simulink model "Riccati_Simulation"  (R2016b)
settings: Solver=VariableStepAuto  StartTime=0.0  StopTime=120  RelTol=1e-1
values from neighbouring files (symbols this model uses):
  A1k = [A1s                     E_w*C_w ... (first row only)    [RiccatiBerechnung_Anlage.m]    (also in RiccatiBerechnunguPlot_Simulation.m)
  A2k = [A2                     E2*C2_s ... (first row only)    [RiccatiBerechnung_Anlage.m]    (also in RiccatiBerechnunguPlot_Simulation.m)
  Ak = [A1                      E*C_s ... (first row only)    [StartSim.m]
  B1 = [0 b2 0 b4]'    [RiccatiBerechnung_Anlage.m]    (also in RiccatiBerechnunguPlot_Simulation.m; StartSim.m)
  B1k = [B1s; zeros(1,size(B1s,2))]    [RiccatiBerechnung_Anlage.m]    (also in RiccatiBerechnunguPlot_Simulation.m)
  B2 = [0  pi*r2*K2/(ue2*T2)]'    [RiccatiBerechnung_Anlage.m]    (also in RiccatiBerechnunguPlot_Simulation.m; StartSim.m = [0  2*pi*r2*K2/(ue2*T2)]')
  B2k = [B2; zeros(1,size(B2,2))]    [RiccatiBerechnung_Anlage.m]    (also in RiccatiBerechnunguPlot_Simulation.m)
  Bk = [B1; zeros(1,size(B1,2))]    [StartSim.m]
  C1k = [C1s [0; 1]]    [RiccatiBerechnung_Anlage.m]    (also in RiccatiBerechnunguPlot_Simulation.m)
  C2k = [C2 zeros(size(C2,1),1)]    [RiccatiBerechnung_Anlage.m]    (also in RiccatiBerechnunguPlot_Simulation.m)
  Ck = [C1 zeros(size(C1,1),1)]    [StartSim.m]
  K1 = 1    [RiccatiBerechnung_Anlage.m]    (also in RiccatiBerechnunguPlot_Simulation.m; StartSim.m)
  K2 = 1    [RiccatiBerechnung_Anlage.m]    (also in RiccatiBerechnunguPlot_Simulation.m; StartSim.m)
  L_0 = 0.5    [RiccatiBerechnunguPlot_Simulation.m]    (also in StartSim.m)
  phi_0 = 0    [RiccatiBerechnunguPlot_Simulation.m]    (also in StartSim.m)
  r1 = 0.0191    [LQG.m]    (also in RiccatiBerechnung_Anlage.m = 0.046; RiccatiBerechnunguPlot_Simulation.m = 0.046; StartSim.m = 0.046)
  R1k = diag([1 30])    [RiccatiBerechnung_Anlage.m]    (also in RiccatiBerechnunguPlot_Simulation.m)
  r2 = 0.015915    [LQG.m]    (also in RiccatiBerechnung_Anlage.m = 0.021975; RiccatiBerechnunguPlot_Simulation.m = 0.021975; StartSim.m = 0.025)
  R2k = 10000    [RiccatiBerechnung_Anlage.m]    (also in RiccatiBerechnunguPlot_Simulation.m)
  T1 = 0.1    [LQG.m]    (also in RiccatiBerechnung_Anlage.m = 0.03032; RiccatiBerechnunguPlot_Simulation.m = 0.03032; StartSim.m = 0.03032)
  T2 = 0.1    [LQG.m]    (also in RiccatiBerechnung_Anlage.m = 0.0247; RiccatiBerechnunguPlot_Simulation.m = 0.0247; StartSim.m = 0.03032)
  ue1 = 6    [RiccatiBerechnung_Anlage.m]    (also in RiccatiBerechnunguPlot_Simulation.m; StartSim.m)
  ue2 = 3    [RiccatiBerechnung_Anlage.m]    (also in RiccatiBerechnunguPlot_Simulation.m; StartSim.m)
  x_0 = 2.54    [RiccatiBerechnunguPlot_Simulation.m]    (also in StartSim.m = 1.3)
undefined symbols (not defined in the file or in its folder): Continuous, K, param, Time
libraries: simulink_extras x4, ctrlSharedLib x2, simulink x1
settings Model: Creator=Patrick  LastModifiedBy=Patrick
settings SolverCC: MaxConsecutiveMinStep=3

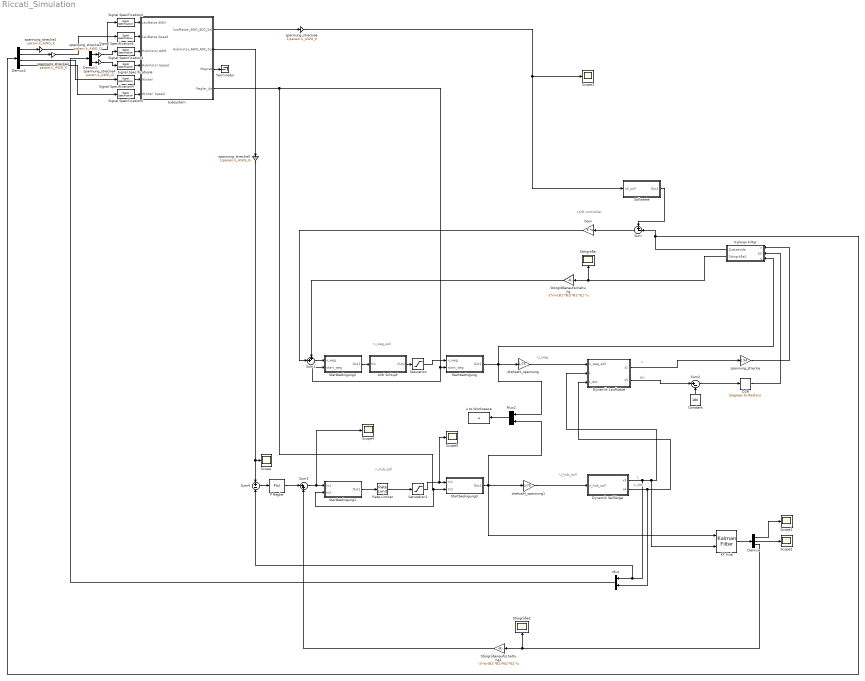
== system Riccati_Simulation ==
  note: L
  note: L_dot
  note: x
  note: psi
  note: LQG controller
  note: U_weg
  note: n_weg_soll
  note: n_hub_soll
  note: U_hub_soll
  Anti Schlupf : Subsystem
  Constant : Constant  Value=180  SampleTime=-1
  D2R : simulink_extras/Transformations/Degrees to Radians
  Demux : Demux  Outputs=3
  Demux1 : Demux  Outputs=2
  Demux2 : Demux
  Dynamik Laufkatze : Subsystem
  Dynamik Seillänge : Subsystem
  Gain : Gain  Gain=K  Multiplication=Matrix(K*u) (u vector)
  KF Hub : ctrlSharedLib/Kalman Filter  TimeDomain=Continuous-Time  UseCurrentEstimator=on  ModelSource=Individual A, B, C, D matrices  ModelSourceVariable=ss(0.95,1,1,0,1)  A=A2k  B=B2k  C=C2k  D=0  NumberOfStates=1  NumberOfInputs=1  NumberOfOutputs=1  InitialEstimateSource=Dialog  X0=0  P0=10  UseK=off  UseGH=on  NumberOfProcessNoiseInputs=1  G=G2k  TimeInvariantG=on  H=0  TimeInvariantH=on  Q=Q2k  TimeInvariantQ=on  R=R2k  TimeInvariantR=on  N=0  TimeInvariantN=on  AddInputPort=on  AddEnablePort=off  ExternalReset=none  OutputEstimatedY=off  OutputP=off  Ts=-1
  Kalman Filter : Subsystem
  Mux : Mux  Inputs=2
  Mux2 : Mux  Inputs=2
  P Regler : simulink/Continuous/PID Controller  Controller=P  TimeDomain=Continuous-time  SampleTime=-1  IntegratorMethod=Forward Euler  FilterMethod=Forward Euler  Form=Parallel  UseFilter=on  ControllerParametersSource=internal  P=25  I=1  D=0  N=100  InitialConditionSource=internal  InitialConditionForIntegrator=0  InitialConditionForFilter=0  ExternalReset=none  LimitOutput=off  UpperSaturationLimit=inf  LowerSaturationLimit=-inf  LinearizeAsGain=on  AntiWindupMode=none  Kb=1  TrackingMode=off  Kt=1  PParamMin=[]  PParamMax=[]  IParamMin=[]  IParamMax=[]  DParamMin=[]  DParamMax=[]  NParamMin=[]  NParamMax=[]  KbParamMin=[]  KbParamMax=[]  KtParamMin=[]  KtParamMax=[]  POutMin=[]  POutMax=[]  IOutMin=[]  IOutMax=[]  DOutMin=[]  DOutMax=[]  NOutMin=[]  NOutMax=[]  KbOutMin=[]  KbOutMax=[]  KtOutMin=[]  KtOutMax=[]  IntegratorOutMin=[]  IntegratorOutMax=[]  FilterOutMin=[]  FilterOutMax=[]  SumOutMin=[]  SumOutMax=[]  SumI1OutMin=[]  SumI1OutMax=[]  SumI2OutMin=[]  SumI2OutMax=[]  SumI3OutMin=[]  SumI3OutMax=[]  SumDOutMin=[]  SumDOutMax=[]  SaturationOutMin=[]  SaturationOutMax=[]  IntegratorContinuousStateAttributes=''  IntegratorStateMustResolveToSignalObject=off  IntegratorRTWStateStorageClass=Auto  FilterContinuousStateAttributes=''  FilterStateMustResolveToSignalObject=off  FilterRTWStateStorageClass=Auto  DifferentiatorICPrevScaledInput=0  DifferentiatorOutMin=[]  DifferentiatorOutMax=[]
  Rate Limiter : RateLimiter  RisingSlewLimit=17  FallingSlewLimit=-17  SampleTimeMode=inherited
  Saturation : Saturate  UpperLimit=75  LowerLimit=-75
  Saturation1 : Saturate  UpperLimit=75  LowerLimit=-75
  Scope{,1..5} (6 alike) : Scope
  Signal Specification{1..6} (6 alike) : SignalSpecification  Dimensions=1
  Sollwerte : Subsystem
  Startbedingung : Subsystem
  Startbedingung1 : Subsystem
  Startbedingung2 : Subsystem
  Startbedingung3 : Subsystem
  Störgröße : Scope
  Störgröße1 : Scope
  Störgrößenaufschaltung : Gain  Gain=-1*inv(B1'*B1)*B1'*E1  Multiplication=Matrix(K*u)
  Störgrößenaufschaltung1 : Gain  Gain=-1*inv(B2'*B2)*B2'*E2  Multiplication=Matrix(K*u)
  Subsystem : Subsystem
  Sum : Sum  Inputs=+-|
  Sum1 : Sum  Inputs=++|
  Sum2 : Sum  Inputs=|+-
  Sum3 : Sum  Inputs=|++
  Sum4 : Sum  Inputs=+-
  Terminator : Terminator
  drehzahl_spannung : Gain  Gain=1/75
  drehzahl_spannung1 : Gain  Gain=1/75
  spannung_strecke : Gain  Gain=2.54
  spannung_strecke1 : Gain  Gain=param.k_AWG_K
  spannung_strecke2 : Gain  Gain=param.k_AWG_K
  spannung_strecke3 : Gain  Gain=param.k_AWG_G
  spannung_strecke4 : Gain  Gain=param.k_AWG_G
  spannung_strecke5 : Gain  Gain=1/param.k_AWG_G
  spannung_strecke6 : Gain  Gain=1/param.k_AWG_K
  u to Workspace : ToWorkspace  VariableName=u  SampleTime=-1
  wires:
  Dynamik Seillänge/2(x4) -> Dynamik Laufkatze/3(L_dot), Mux/2
  Mux2/1 -> u to Workspace/1
  Sum/1 -> Gain/1
  Gain/1 -> Sum1/2
  Dynamik Laufkatze/1(x1) -> spannung_strecke/1
  drehzahl_spannung/1 -> Dynamik Laufkatze/1(n_weg_soll)
  Anti Schlupf/1(Out1) -> Saturation/1
  Kalman Filter/2(Störgröße1) -> Störgrößenaufschaltung/1, Störgröße/1
  spannung_strecke/1 -> Kalman Filter/1(x)
  D2R/1 -> Kalman Filter/2(psi)
  Störgrößenaufschaltung/1 -> Sum1/1
  Dynamik Laufkatze/2(x5) -> Sum2/1
  Constant/1 -> Sum2/2
  Startbedingung/1(Out1) -> Mux2/1, drehzahl_spannung/1, Kalman Filter/3(u)
  Subsystem/4(Regler_An) -> Startbedingung1/2(In2), Startbedingung3/2(In2), Startbedingung2/2(start_weg), Startbedingung/2(start_weg)
  Sollwerte/1(Out1) -> Sum/1
  Startbedingung1/1(Out1) -> Rate Limiter/1
  Saturation/1 -> Startbedingung/1(x_weg)
  Sum2/1 -> D2R/1
  Sum1/1 -> Startbedingung2/1(x_weg)
  Startbedingung2/1(Out1) -> Anti Schlupf/1(In1)
  KF Hub/1 -> Demux/1
  Demux/3 -> Störgröße1/1, Störgrößenaufschaltung1/1
  Rate Limiter/1 -> Saturation1/1
  Saturation1/1 -> Scope5/1, Startbedingung3/1(In1)
  Startbedingung3/1(Out1) -> drehzahl_spannung1/1, KF Hub/1, Mux2/2
  Demux/1 -> Scope1/1
  Demux/2 -> Scope2/1
  Mux/1 -> Demux1/1
  Kalman Filter/1(Zustaende) -> Demux2/1, Sum/2
  Dynamik Seillänge/1(x3) -> Dynamik Laufkatze/2(L), KF Hub/2, Sum4/2, Mux/1
  P Regler/1 -> Sum3/1
  Sum3/1 -> Scope4/1, Startbedingung1/1(In1)
  Störgrößenaufschaltung1/1 -> Sum3/2
  Demux1/1 -> spannung_strecke3/1
  Demux1/2 -> spannung_strecke4/1
  Demux2/1 -> spannung_strecke1/1
  Demux2/2 -> spannung_strecke2/1
  Demux2/3 -> Signal Specification4/1
  Demux2/4 -> Signal Specification5/1
  Subsystem/1(Laufkatze_AWG_ADC_Soll) -> spannung_strecke6/1
  Signal Specification2/1 -> Subsystem/1(Laufkatze AWG)
  Signal Specification1/1 -> Subsystem/2(Laufkatze Speed)
  Signal Specification3/1 -> Subsystem/3(Hubmotor AWG)
  Signal Specification4/1 -> Subsystem/5(Winkel)
  Signal Specification5/1 -> Subsystem/6(Winkel  Speed)
  Signal Specification6/1 -> Subsystem/4(Hubmotor Speed)
  Subsystem/3(Magnet) -> Terminator/1
  spannung_strecke1/1 -> Signal Specification2/1
  spannung_strecke2/1 -> Signal Specification1/1
  spannung_strecke3/1 -> Signal Specification3/1
  spannung_strecke4/1 -> Signal Specification6/1
  Subsystem/2(Hubmotor_AWG_ADC_Soll) -> spannung_strecke5/1
  spannung_strecke6/1 -> Scope3/1, Sollwerte/1(x1_soll)
  Sum4/1 -> P Regler/1
  spannung_strecke5/1 -> Sum4/1, Scope/1
  drehzahl_spannung1/1 -> Dynamik Seillänge/1(n_hub_soll)

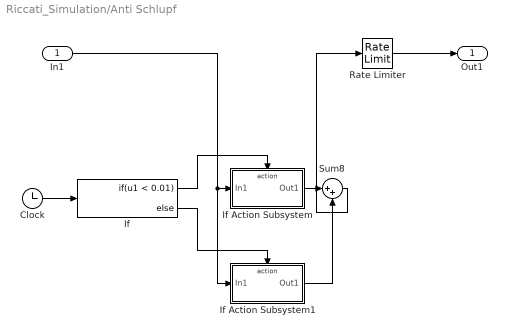
== system Riccati_Simulation/Anti Schlupf ==
  In1 : Inport
  Clock : Clock
  If : If  IfExpression=u1 < 0.01
  If Action Subsystem : Subsystem  TreatAsAtomicUnit=on
  If Action Subsystem1 : Subsystem  TreatAsAtomicUnit=on
  Rate Limiter : RateLimiter  RisingSlewLimit=9.57  FallingSlewLimit=-9.57  SampleTimeMode=inherited
  Sum8 : Sum  Inputs=|++
  Out1 : Outport
  wires:
  In1/1 -> If Action Subsystem1/1(In1), If Action Subsystem/1(In1)
  If Action Subsystem/1(Out1) -> Sum8/1
  If Action Subsystem1/1(Out1) -> Sum8/2
  Sum8/1 -> Rate Limiter/1
  If/1 -> If Action Subsystem/Action
  If/2 -> If Action Subsystem1/Action
  Rate Limiter/1 -> Out1/1
  Clock/1 -> If/1

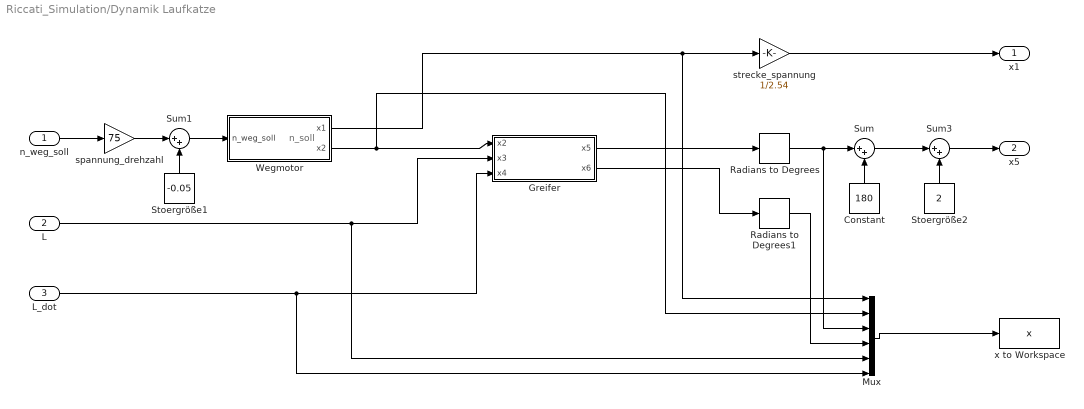
== system Riccati_Simulation/Dynamik Laufkatze ==
  note: n_soll
  n_weg_soll : Inport
  L : Inport  Port=2
  L_dot : Inport  Port=3
  Constant : Constant  Value=180  SampleTime=-1
  Greifer : Subsystem
  Mux : Mux  Inputs=6
  Radians to Degrees : simulink_extras/Transformations/Radians to Degrees
  Radians to Degrees1 : simulink_extras/Transformations/Radians to Degrees
  Stoergröße1 : Constant  Value=-0.05  SampleTime=-1
  Stoergröße2 : Constant  Value=2  SampleTime=-1
  Sum : Sum  Inputs=|++
  Sum1 : Sum  Inputs=|++
  Sum3 : Sum  Inputs=|++
  Wegmotor : Subsystem
  spannung_drehzahl : Gain  Gain=75
  strecke_spannung : Gain  Gain=1/2.54
  x to Workspace : ToWorkspace  VariableName=x  SampleTime=-1
  x1 : Outport
  x5 : Outport  Port=2
  wires:
  Wegmotor/2(x2) -> Mux/2, Greifer/1(x2)
  Greifer/2(x6) -> Radians to Degrees1/1
  L/1 -> Mux/5, Greifer/2(x3)
  L_dot/1 -> Mux/6, Greifer/3(x4)
  Radians to Degrees1/1 -> Mux/4
  Mux/1 -> x to Workspace/1
  strecke_spannung/1 -> x1/1
  Wegmotor/1(x1) -> strecke_spannung/1, Mux/1
  Sum3/1 -> x5/1
  Radians to Degrees/1 -> Mux/3, Sum/1
  Sum/1 -> Sum3/1
  Constant/1 -> Sum/2
  n_weg_soll/1 -> spannung_drehzahl/1
  Stoergröße1/1 -> Sum1/2
  Sum1/1 -> Wegmotor/1(n_weg_soll)
  spannung_drehzahl/1 -> Sum1/1
  Greifer/1(x5) -> Radians to Degrees/1
  Stoergröße2/1 -> Sum3/2

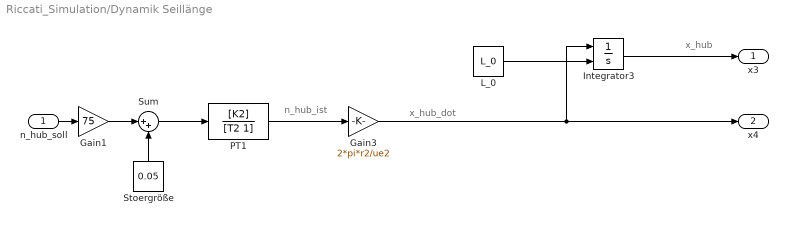
== system Riccati_Simulation/Dynamik Seillänge ==
  note: n_hub_ist
  note: x_hub_dot
  note: x_hub
  n_hub_soll : Inport
  Gain1 : Gain  Gain=75
  Gain3 : Gain  Gain=2*pi*r2/ue2
  Integrator3 : Integrator  InitialConditionSource=external
  L_0 : Constant  Value=L_0  SampleTime=-1
  PT1 : TransferFcn  Numerator=[K2]  Denominator=[T2 1]
  Stoergröße : Constant  Value=0.05  SampleTime=-1
  Sum : Sum  Inputs=|++
  x3 : Outport
  x4 : Outport  Port=2
  wires:
  n_hub_soll/1 -> Gain1/1
  PT1/1 -> Gain3/1
  Integrator3/1 -> x3/1
  L_0/1 -> Integrator3/2
  Gain3/1 -> Integrator3/1, x4/1
  Sum/1 -> PT1/1
  Gain1/1 -> Sum/1
  Stoergröße/1 -> Sum/2

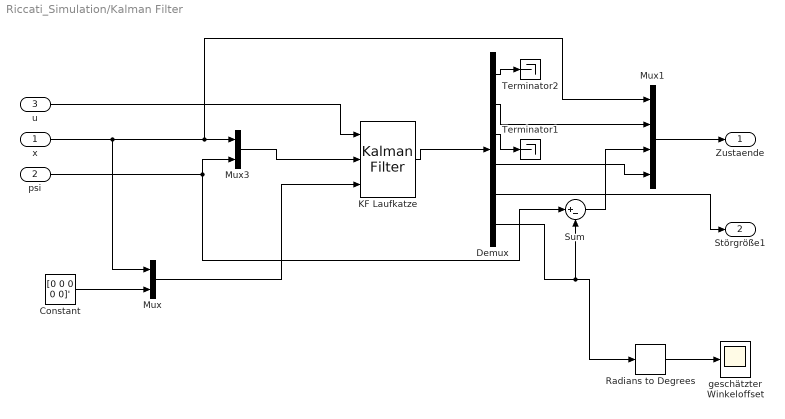
== system Riccati_Simulation/Kalman Filter ==
  x : Inport
  psi : Inport  Port=2
  u : Inport  Port=3
  Constant : Constant  Value=[0 0 0 0 0]'
  Demux : Demux  Outputs=6
  KF Laufkatze : ctrlSharedLib/Kalman Filter  TimeDomain=Continuous-Time  UseCurrentEstimator=on  ModelSource=Individual A, B, C, D matrices  ModelSourceVariable=ss(Ak,Bk,Ck,0)  A=A1k  B=B1k  C=C1k  D=0  NumberOfStates=1  NumberOfInputs=1  NumberOfOutputs=1  InitialEstimateSource=Input port  X0=0  P0=10  UseK=off  UseGH=on  NumberOfProcessNoiseInputs=1  G=G1k  TimeInvariantG=on  H=0  TimeInvariantH=on  Q=Q1k  TimeInvariantQ=on  R=R1k  TimeInvariantR=on  N=0  TimeInvariantN=on  AddInputPort=on  AddEnablePort=off  ExternalReset=none  OutputEstimatedY=off  OutputP=off  Ts=-1
  Mux : Mux  Inputs=2
  Mux1 : Mux
  Mux3 : Mux  Inputs=2
  Radians to Degrees : simulink_extras/Transformations/Radians to Degrees
  Sum : Sum  Inputs=|+-
  Terminator1 : Terminator
  Terminator2 : Terminator
  geschätzter Winkeloffset : Scope
  Zustaende : Outport
  Störgröße1 : Outport  Port=2
  wires:
  KF Laufkatze/1 -> Demux/1
  psi/1 -> Sum/1, Mux3/2
  x/1 -> Mux/1, Mux1/1, Mux3/1
  u/1 -> KF Laufkatze/1
  Demux/2 -> Mux1/2
  Demux/4 -> Mux1/4
  Mux1/1 -> Zustaende/1
  Demux/5 -> Störgröße1/1
  Demux/1 -> Terminator2/1
  Demux/3 -> Terminator1/1
  Mux3/1 -> KF Laufkatze/2
  Constant/1 -> Mux/2
  Mux/1 -> KF Laufkatze/3
  Demux/6 -> Radians to Degrees/1, Sum/2
  Sum/1 -> Mux1/3
  Radians to Degrees/1 -> geschätzter Winkeloffset/1

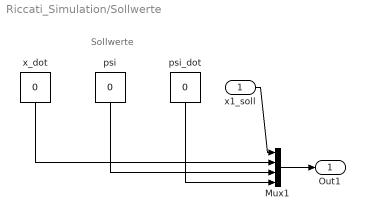
== system Riccati_Simulation/Sollwerte ==
  note: Sollwerte
  x1_soll : Inport
  Mux1 : Mux
  psi : Constant  Value=0
  psi_dot : Constant  Value=0
  x_dot : Constant  Value=0
  Out1 : Outport
  wires:
  psi_dot/1 -> Mux1/4
  x_dot/1 -> Mux1/2
  psi/1 -> Mux1/3
  Mux1/1 -> Out1/1
  x1_soll/1 -> Mux1/1

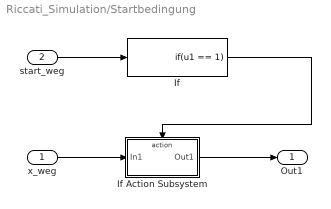
== system Riccati_Simulation/Startbedingung ==
  x_weg : Inport
  start_weg : Inport  Port=2
  If : If  IfExpression=u1 == 1  ShowElse=off
  If Action Subsystem : Subsystem  TreatAsAtomicUnit=on
  Out1 : Outport
  wires:
  If Action Subsystem/1(Out1) -> Out1/1
  x_weg/1 -> If Action Subsystem/1(In1)
  start_weg/1 -> If/1
  If/1 -> If Action Subsystem/Action

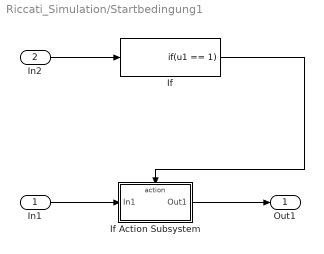
== system Riccati_Simulation/Startbedingung1 ==
  In1 : Inport
  In2 : Inport  Port=2
  If : If  IfExpression=u1 == 1  ShowElse=off
  If Action Subsystem : Subsystem  TreatAsAtomicUnit=on
  Out1 : Outport
  wires:
  If Action Subsystem/1(Out1) -> Out1/1
  In1/1 -> If Action Subsystem/1(In1)
  In2/1 -> If/1
  If/1 -> If Action Subsystem/Action

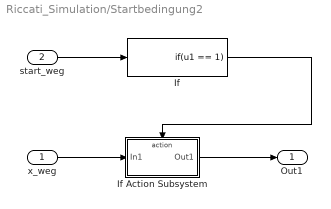
== system Riccati_Simulation/Startbedingung2 ==
  x_weg : Inport
  start_weg : Inport  Port=2
  If : If  IfExpression=u1 == 1  ShowElse=off
  If Action Subsystem : Subsystem  TreatAsAtomicUnit=on
  Out1 : Outport
  wires:
  If Action Subsystem/1(Out1) -> Out1/1
  x_weg/1 -> If Action Subsystem/1(In1)
  start_weg/1 -> If/1
  If/1 -> If Action Subsystem/Action

== system Riccati_Simulation/Startbedingung3 ==
  In1 : Inport
  In2 : Inport  Port=2
  If : If  IfExpression=u1 == 1  ShowElse=off
  If Action Subsystem : Subsystem  TreatAsAtomicUnit=on
  Out1 : Outport
  wires:
  If Action Subsystem/1(Out1) -> Out1/1
  In1/1 -> If Action Subsystem/1(In1)
  In2/1 -> If/1
  If/1 -> If Action Subsystem/Action

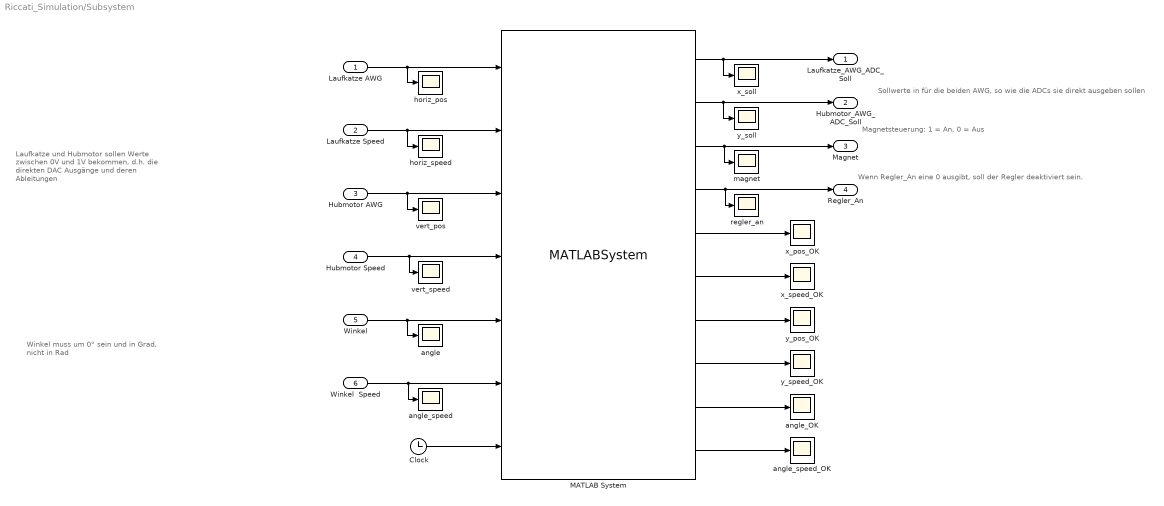
== system Riccati_Simulation/Subsystem ==
  note: Winkel muss um 0° sein und in Grad,
      | nicht in Rad
  note: Magnetsteuerung: 1 = An, 0 = Aus
  note: Sollwerte in für die beiden AWG, so wie die ADCs sie direkt ausgeben sollen
  note: Wenn Regler_An eine 0 ausgibt, soll der Regler deaktiviert sein.
  note: Laufkatze und Hubmotor sollen
      | Werte zwischen 0V und 1V bekommen,
      | d.h. die direkten DAC Ausgänge und
      | deren Ableitungen
  Laufkatze AWG : Inport  OutMin=0  OutMax=1  OutDataTypeStr=double  PortDimensions=1
  Laufkatze Speed : Inport  Port=2  OutDataTypeStr=double
  Hubmotor AWG : Inport  Port=3  OutMin=0  OutMax=1  OutDataTypeStr=double  PortDimensions=1
  Hubmotor Speed : Inport  Port=4  OutDataTypeStr=double
  Winkel : Inport  Port=5  OutMin=0  OutMax=360  OutDataTypeStr=double  PortDimensions=1
  Winkel  Speed : Inport  Port=6  OutDataTypeStr=double
  Clock : Clock
  MATLAB System : MATLABSystem  System=Steuerung_Automatisierung  start_time=10  add_midpoints=true  midpoint_height=35  param=param  SimulateUsing=Code generation
      mask Type: Steuerung_Automatisierung
      mask Display:
      | disp('Steuerung_Automatisierung');
      | port_label('input',1,'horiz_pos');
      | port_label('input',2,'horiz_speed');
      | port_label('input',3,'vert_pos');
      | port_label('input',4,'vert_speed');
      | port_label('input',5,'angle');
      | port_label('input',6,'angle_speed');
      | port_label('input',7,'Clock');
      | port_label('output',1,'horiz_setpoint');
      | port_label('output',2,'vert_setpoint');
      | port_label('output',3,'magnet_on');
      | port_label('output',4,'control_enable');
      | port_label('output',5,'x_under_thres');
      | port_label('output',6,'x_speed_under_thres');
      | port_label('output',7,'y_under_thres');
      | port_label('output',8,'y_speed_under_thres');
      | port_label('output',9,'angle_under_thres');
      | port_label('output',10,'angle_speed_under_thres');
  angle : Scope
  angle_OK : Scope
  angle_speed : Scope
  angle_speed_OK : Scope
  horiz_pos : Scope
  horiz_speed : Scope
  magnet : Scope
  regler_an : Scope
  vert_pos : Scope
  vert_speed : Scope
  x_pos_OK : Scope
  x_soll : Scope
  x_speed_OK : Scope
  y_pos_OK : Scope
  y_soll : Scope
  y_speed_OK : Scope
  Laufkatze_AWG_ADC_Soll : Outport
  Hubmotor_AWG_ADC_Soll : Outport  Port=2
  Magnet : Outport  Port=3
  Regler_An : Outport  Port=4
  wires:
  Laufkatze AWG/1 -> MATLAB System/1, horiz_pos/1
  Hubmotor AWG/1 -> MATLAB System/3, vert_pos/1
  Winkel/1 -> MATLAB System/5, angle/1
  MATLAB System/4 -> regler_an/1, Regler_An/1
  MATLAB System/1 -> x_soll/1, Laufkatze_AWG_ADC_Soll/1
  MATLAB System/3 -> Magnet/1, magnet/1
  Clock/1 -> MATLAB System/7
  MATLAB System/2 -> y_soll/1, Hubmotor_AWG_ADC_Soll/1
  MATLAB System/5 -> x_pos_OK/1
  MATLAB System/6 -> x_speed_OK/1
  MATLAB System/7 -> y_pos_OK/1
  MATLAB System/8 -> y_speed_OK/1
  MATLAB System/9 -> angle_OK/1
  MATLAB System/10 -> angle_speed_OK/1
  Laufkatze Speed/1 -> MATLAB System/2, horiz_speed/1
  Hubmotor Speed/1 -> MATLAB System/4, vert_speed/1
  Winkel  Speed/1 -> MATLAB System/6, angle_speed/1

== system Riccati_Simulation/Anti Schlupf/If Action Subsystem ==
  In1 : Inport
  Action Port : ActionPort  ActionType=then
  Gain : Gain  Gain=0
  Out1 : Outport
  wires:
  In1/1 -> Gain/1
  Gain/1 -> Out1/1

== system Riccati_Simulation/Anti Schlupf/If Action Subsystem1 ==
  In1 : Inport
  Action Port : ActionPort  ActionType=else
  Gain : Gain
  Out1 : Outport
  wires:
  In1/1 -> Gain/1
  Gain/1 -> Out1/1

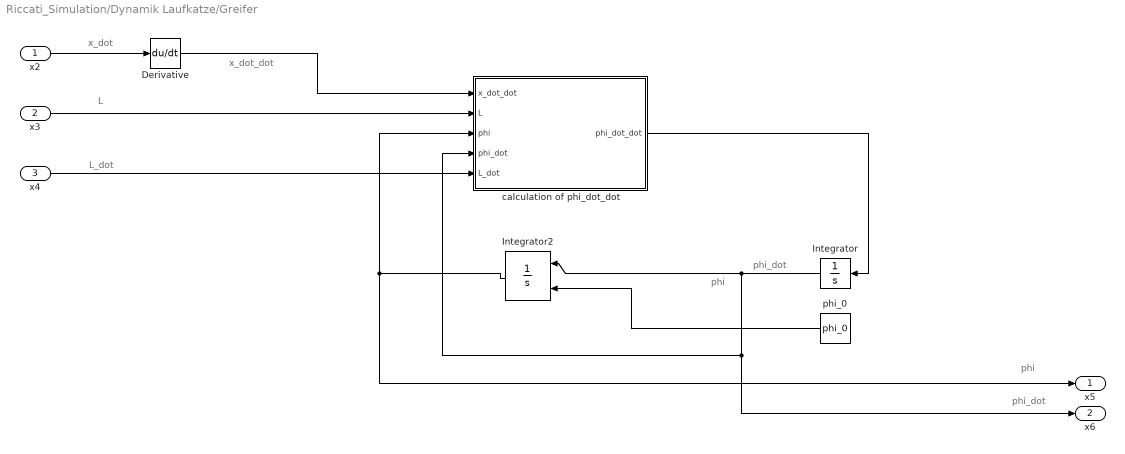
== system Riccati_Simulation/Dynamik Laufkatze/Greifer ==
  note: phi
  note: phi
  note: x_dot
  note: L
  note: phi_dot
  note: phi_dot
  note: x_dot_dot
  note: L_dot
  x2 : Inport
  x3 : Inport  Port=2
  x4 : Inport  Port=3
  Derivative : Derivative
  Integrator : Integrator
  Integrator2 : Integrator  InitialConditionSource=external
  calculation of phi_dot_dot : MATLAB Function  TreatAsAtomicUnit=on
  phi_0 : Constant  Value=phi_0  SampleTime=-1
  x5 : Outport
  x6 : Outport  Port=2
  wires:
  Derivative/1 -> calculation of phi_dot_dot/1(x_dot_dot)
  x2/1 -> Derivative/1
  Integrator/1 -> x6/1, calculation of phi_dot_dot/4(phi_dot), Integrator2/1
  x3/1 -> calculation of phi_dot_dot/2(L)
  calculation of phi_dot_dot/1(phi_dot_dot) -> Integrator/1
  Integrator2/1 -> x5/1, calculation of phi_dot_dot/3(phi)
  x4/1 -> calculation of phi_dot_dot/5(L_dot)
  phi_0/1 -> Integrator2/2

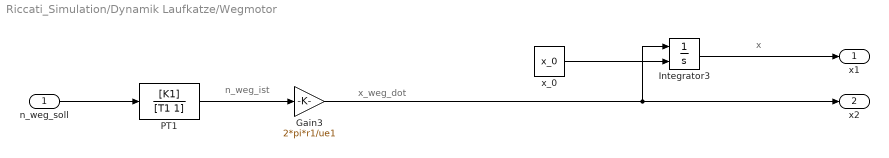
== system Riccati_Simulation/Dynamik Laufkatze/Wegmotor ==
  note: n_weg_ist
  note: x
  note: x_weg_dot
  n_weg_soll : Inport
  Gain3 : Gain  Gain=2*pi*r1/ue1
  Integrator3 : Integrator  InitialConditionSource=external
  PT1 : TransferFcn  Numerator=[K1]  Denominator=[T1 1]
  x_0 : Constant  Value=x_0  SampleTime=-1
  x1 : Outport
  x2 : Outport  Port=2
  wires:
  x_0/1 -> Integrator3/2
  n_weg_soll/1 -> PT1/1
  PT1/1 -> Gain3/1
  Integrator3/1 -> x1/1
  Gain3/1 -> Integrator3/1, x2/1

== system Riccati_Simulation/Startbedingung/If Action Subsystem ==
  In1 : Inport
  Action Port : ActionPort  ActionType=then
  Out1 : Outport
  wires:
  In1/1 -> Out1/1

== system Riccati_Simulation/Startbedingung1/If Action Subsystem ==
  In1 : Inport
  Action Port : ActionPort  ActionType=then
  Out1 : Outport
  wires:
  In1/1 -> Out1/1

== system Riccati_Simulation/Startbedingung2/If Action Subsystem ==
  In1 : Inport
  Action Port : ActionPort  ActionType=then
  Out1 : Outport
  wires:
  In1/1 -> Out1/1

== system Riccati_Simulation/Startbedingung3/If Action Subsystem ==
  In1 : Inport
  Action Port : ActionPort  ActionType=then
  Out1 : Outport
  wires:
  In1/1 -> Out1/1

== matlab function Riccati_Simulation/Dynamik Laufkatze/Greifer/calculation of phi_dot_dot ==
  data: x_dot_dot input; phi_dot_dot output; L input; phi input; phi_dot input; L_dot input
function phi_dot_dot = fcn(x_dot_dot,L,phi,phi_dot,L_dot)

phi_dot_dot = -(cos(phi)/L)*x_dot_dot-9.81/L*sin(phi)-2*L_dot*phi_dot;
